simulink model "untitled"  (R2022a)
settings: Solver=VariableStepAuto  StartTime=0.0  StopTime=10.0  RelTol=1e-3
settings Model: Creator=darre  LastModifiedBy=Darren Au
settings DebuggingCC: UnconnectedInputMsg=warning  UnconnectedOutputMsg=warning  UnconnectedLineMsg=warning
settings RTWCC: DLArmComputeVersion=19.05

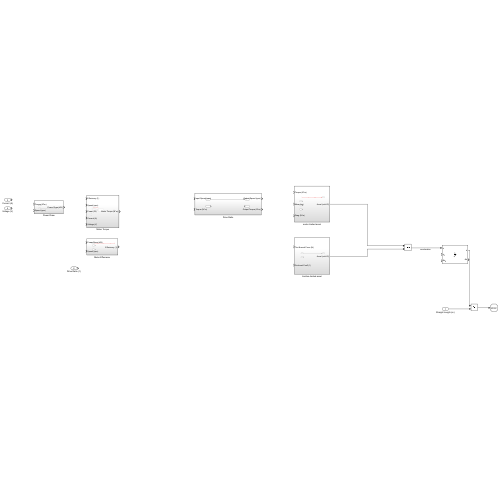
[thumbnail: Simulink's stored preview of the top-level diagram]
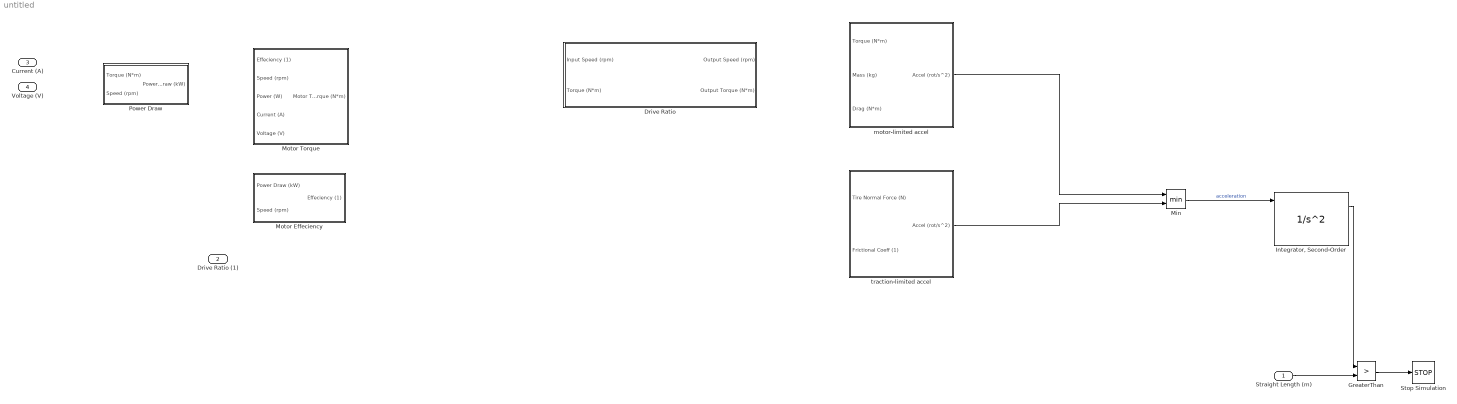
== system untitled ==
  Straight Length (m) : Inport
  Drive Ratio (1) : Inport  Port=2
  Current (A) : Inport  Port=3
  Voltage (V) : Inport  Port=4
  Drive Ratio : Subsystem
  GreaterThan : RelationalOperator  Operator=>  OutDataTypeStr=boolean  RndMeth=Simplest  InputSameDT=off
  "Integrator, Second-Order" : SecondOrderIntegrator  ICSourceX=external  ICSourceDXDT=external
  Min : MinMax  Inputs=2
  Motor Effeciency : Subsystem
  Motor Torque : Subsystem
  Power Draw : Subsystem
  Stop Simulation : Stop
  motor-limited accel : Subsystem
  traction-limited accel : Subsystem
  wires:
  Min/1 -> "Integrator, Second-Order"/1  "acceleration"
  "Integrator, Second-Order"/1 -> GreaterThan/1
  Straight Length (m)/1 -> GreaterThan/2
  GreaterThan/1 -> Stop Simulation/1
  motor-limited accel/1(Accel (rot/s^2)) -> Min/1
  traction-limited accel/1(Accel (rot/s^2)) -> Min/2

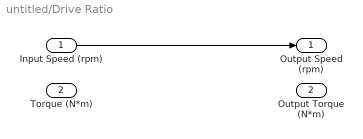
== system untitled/Drive Ratio ==
  Input Speed (rpm) : Inport
  Torque (N*m) : Inport  Port=2
  Output Speed (rpm) : Outport
  Output Torque (N*m) : Outport  Port=2
  wires:
  Input Speed (rpm)/1 -> Output Speed (rpm)/1

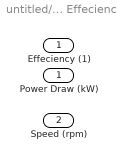
== system untitled/Motor Effeciency ==
  Power Draw (kW) : Inport
  Speed (rpm) : Inport  Port=2
  Effeciency (1) : Outport
  wires:
  ? -> ?

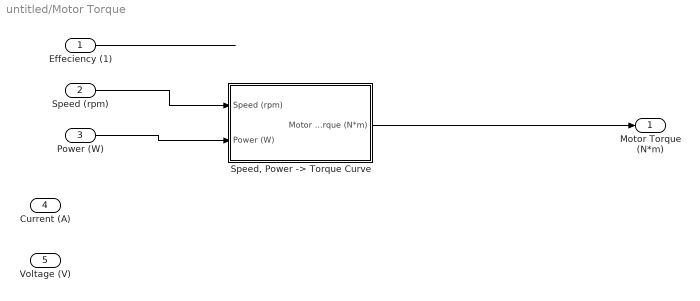
== system untitled/Motor Torque ==
  Effeciency (1) : Inport
  Speed (rpm) : Inport  Port=2
  Power (W) : Inport  Port=3
  Current (A) : Inport  Port=4
  Voltage (V) : Inport  Port=5
  "Speed, Power -> Torque Curve" : Subsystem
  Motor Torque (N*m) : Outport
  wires:
  Effeciency (1)/1 -> ?
  Speed (rpm)/1 -> "Speed, Power -> Torque Curve"/1(Speed (rpm))
  Power (W)/1 -> "Speed, Power -> Torque Curve"/2(Power (W))
  "Speed, Power -> Torque Curve"/1(Motor Torque (N*m)) -> Motor Torque (N*m)/1

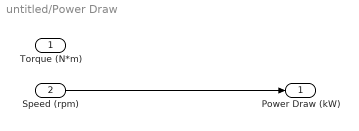
== system untitled/Power Draw ==
  Torque (N*m) : Inport
  Speed (rpm) : Inport  Port=2
  Power Draw (kW) : Outport
  wires:
  Speed (rpm)/1 -> Power Draw (kW)/1

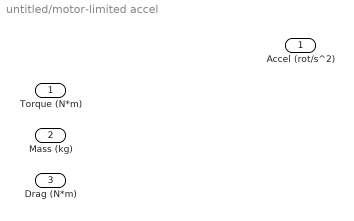
== system untitled/motor-limited accel ==
  Torque (N*m) : Inport
  Mass (kg) : Inport  Port=2
  Drag (N*m) : Inport  Port=3
  Accel (rot/s^2) : Outport
  wires:
  ? -> Accel (rot/s^2)/1

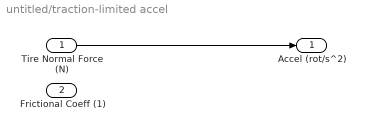
== system untitled/traction-limited accel ==
  Tire Normal Force (N) : Inport
  Frictional Coeff (1) : Inport  Port=2
  Accel (rot/s^2) : Outport
  wires:
  Tire Normal Force (N)/1 -> Accel (rot/s^2)/1

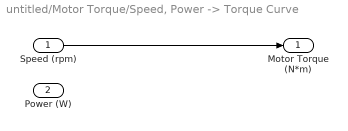
== system untitled/Motor Torque/Speed, Power -> Torque Curve ==
  Speed (rpm) : Inport
  Power (W) : Inport  Port=2
  Motor Torque (N*m) : Outport
  wires:
  Speed (rpm)/1 -> Motor Torque (N*m)/1
